simulink model "TestBlock"  (R2018a)
settings: Solver=VariableStepAuto  StartTime=0.0  StopTime=60  RelTol=1e-3
settings Model: Creator=rashe  LastModifiedBy=rashe

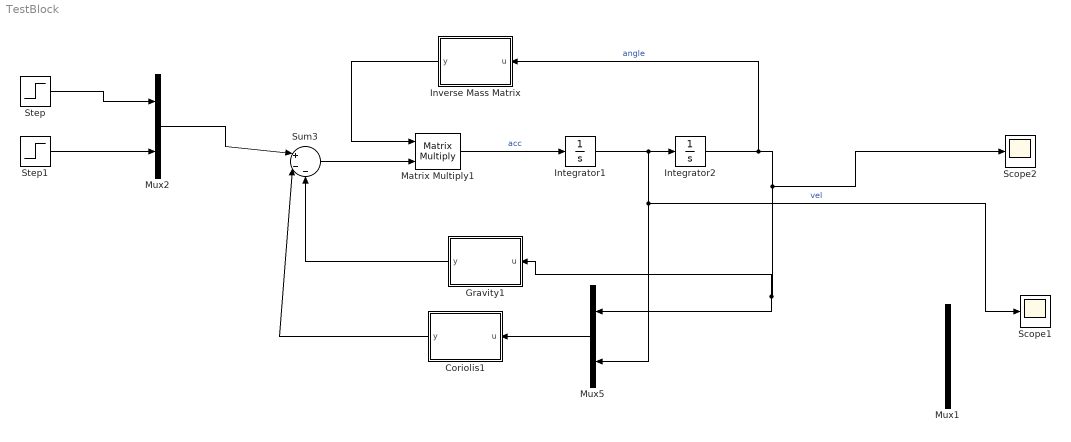
== system TestBlock ==
  Coriolis1 : MATLAB Function  TreatAsAtomicUnit=on
  Gravity1 : MATLAB Function  TreatAsAtomicUnit=on
  Integrator1 : Integrator  InitialCondition=[0; 0]
  Integrator2 : Integrator  InitialCondition=[0; 0]
  Inverse Mass Matrix : MATLAB Function  TreatAsAtomicUnit=on
  Matrix Multiply1 : Product  Multiplication=Matrix(*)
  Mux1 : Mux  Inputs=2
  Mux2 : Mux  Inputs=2
  Mux5 : Mux  Inputs=2
  Scope1 : Scope
  Scope2 : Scope
  Step : Step  After=0  SampleTime=0
  Step1 : Step  Time=2  After=0.0001  SampleTime=0
  Sum3 : Sum  Inputs=|+--
  wires:
  Inverse Mass Matrix/1(y) -> Matrix Multiply1/1
  Integrator1/1 -> Scope1/1, Mux5/2, Integrator2/1  "vel"
  Sum3/1 -> Matrix Multiply1/2
  Coriolis1/1(y) -> Sum3/2
  Gravity1/1(y) -> Sum3/3
  Mux5/1 -> Coriolis1/1(u)
  Matrix Multiply1/1 -> Integrator1/1  "acc"
  Integrator2/1 -> Scope2/1, Mux5/1, Gravity1/1(u), Inverse Mass Matrix/1(u)  "angle"
  Mux2/1 -> Sum3/1
  Step/1 -> Mux2/1
  Step1/1 -> Mux2/2

== matlab function TestBlock/Inverse Mass Matrix ==
  data: u input; y output
function y = INVMass(u)

the1 = u(1);
the2 = u(2);

m1 = 0.233;   %kg
m2 = 0.2;
l1 = 0.192;
l2 = 0.185;
L1 = 0.27;
L2 = 0.23;
g = 9.81;

I1 = (1/3)*m1*l1^2;
I2 = (1/3)*m2*l2^2;

M11 = m1*l1^2 + m2*(L1^2 + l2^2 + L1*l2*cos(the2)) + I1 + I2;
M12 = m2*(l2^2 + L1*l2*cos(the2)) + I2;
M21 = m2*(l2^2 + L1*l2*cos(the2)) + I2;
M22 = m2*l2^2 + I2;

coef = 1/(M11*M22 - M12*M21);
invM = coef*[M22, -M12; -M21, M11];

y = invM;

== matlab function TestBlock/Coriolis1 ==
  data: u input; y output
function y = V(u)

the1 = u(1);
the2 = u(2);

vel1 = u(3);
vel2 = u(4);

m1 = 0.233;   %kg
m2 = 0.2;
l1 = 0.192;
l2 = 0.185;
L1 = 0.27;
L2 = 0.23;
g = 9.81;

I1 = (1/3)*m1*l1^2;
I2 = (1/3)*m2*l2^2;


V11 = -m2*L1*l2*sin(the2)*(vel1*vel2 + 0.5*vel2^2);
V21 = 0.5*m2*L1*l2*sin(the2)*vel1^2;


y = [V11;V21];

== matlab function TestBlock/Gravity1 ==
  data: u input; y output
function y = G(u)

the1 = u(1);
the2 = u(2);

m1 = 0.233;   %kg
m2 = 0.2;
l1 = 0.192;
l2 = 0.185;
L1 = 0.27;
L2 = 0.23;
g = 9.81;

I1 = (1/3)*m1*l1^2;
I2 = (1/3)*m2*l2^2;

G11 = m1*g*l1*cos(the1) + m2*g*L1*cos(the1) + m2*g*l2*cos(the1+the2);
G21 = m2*g*l2*cos(the1+the2);

y = [G11;G21];
